simulink model "Chevrolet_PHEVmodel"  (R2024b)
settings: Solver=VariableStepAuto  StartTime=0.0  StopTime=10.0  RelTol=1e-3
undefined symbols (not defined in the file): automatic_gearbox, DiscIntNeverNeededParam, eta_EG_map, eta_EM_map, g, h, H_u, k_cs, P_aux, P_CE_cutoff, P_CE_idle, r, rho, rho_f, T_CE_cutoff, T_CE_max, T_EG_max, T_EM_max, theta_CE, theta_EM, V_CE_map, w_CE_idle, w_CE_max, w_CE_upper, w_EG_row, w_EG_upper, w_EM_row, w_EM_upper
(part 1 of 2)
settings Model: Creator=Imane  LastModifiedBy=Imane

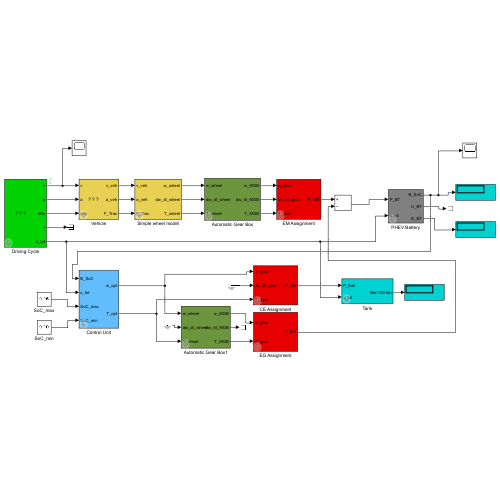
[thumbnail: Simulink's stored preview of the top-level diagram]
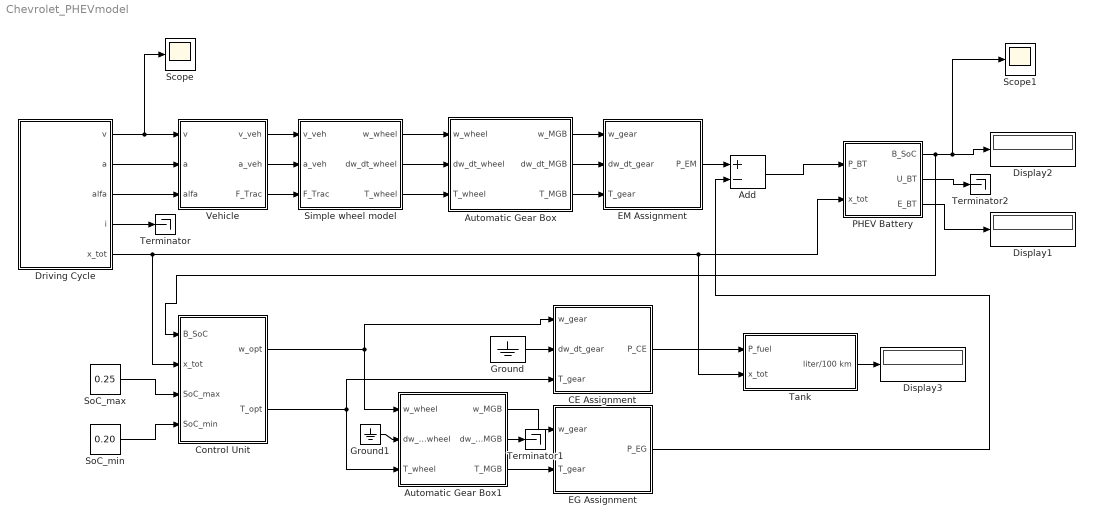
== system Chevrolet_PHEVmodel ==
  Add : Sum  Inputs=+-
  Automatic Gear Box : Subsystem  Tag=transmission  mask(Automatic Gear Box){nog=1, i=[1], i_diff=5, gearon=[], gearoff=[], d=0.62, e_GT=0.98, P_GT0=300, w_wheel_min=1}
      mask prompts: nog "Number of gears"; i "Gear ratio vector"; i_diff "Differential gear [-]"; gearon "Switching points for upshift [km/h]"; gearoff "Switching points for downshift [km/h]"; d "Wheel diameter"; e_GT "Efficiency [-]"; P_GT0 "Idling losses (friction) [W]"; w_wheel_min "Minimum wheel speed beyond which losses are generated [rad/s]"
      mask help:
      | This block simulates a automatic gear box, can handle up to 16 gears.
      |
      | Input:
      | =====
      | 	w_wheel	Speed of the wheel [rad/s]
      | 	dw_dt_wheel	Acceleration of the wheel [rad/s^2],
      | 	T_wheel	Torque on the wheel [Nm]
      | 	i	Gear number [-]
      |
      | Output:
      | ======
      | 	w_MGB	Speed of the fly wheel [rad/s]
      | 	dw_dt_MGB	Acceleration of the fly wheel [rad/s^2]
      | 	T_MGB	Torque on the fly wheel [Nm]
      |
      | Number of gears:
      | ======
      | Specify the number of forward gears
      |
      | Shifting points for upshift:
      | ======
      | Vector specifying the velocity for shifting
      | [first_to_second_gear    second_to_third_gear    ....]
      | The number of elements in the vector should be Number of gears - 1.
      |
      | Shifting points for udownshift:
      | ======
      | Simular to upshift
      | [second_to_first_gear    third_to_second_gear    ....]
      mask init:
      | init_AGB;
  Automatic Gear Box1 : Subsystem  Tag=transmission  mask(Automatic Gear Box){nog=1, i=[1], i_diff=1, gearon=[], gearoff=[], d=0.62, e_GT=0.98, P_GT0=0, w_wheel_min=1}
      mask prompts: nog "Number of gears"; i "Gear ratio vector"; i_diff "Differential gear [-]"; gearon "Switching points for upshift [km/h]"; gearoff "Switching points for downshift [km/h]"; d "Wheel diameter"; e_GT "Efficiency [-]"; P_GT0 "Idling losses (friction) [W]"; w_wheel_min "Minimum wheel speed beyond which losses are generated [rad/s]"
      mask help:
      | This block simulates a automatic gear box, can handle up to 16 gears.
      |
      | Input:
      | =====
      | 	w_wheel	Speed of the wheel [rad/s]
      | 	dw_dt_wheel	Acceleration of the wheel [rad/s^2],
      | 	T_wheel	Torque on the wheel [Nm]
      | 	i	Gear number [-]
      |
      | Output:
      | ======
      | 	w_MGB	Speed of the fly wheel [rad/s]
      | 	dw_dt_MGB	Acceleration of the fly wheel [rad/s^2]
      | 	T_MGB	Torque on the fly wheel [Nm]
      |
      | Number of gears:
      | ======
      | Specify the number of forward gears
      |
      | Shifting points for upshift:
      | ======
      | Vector specifying the velocity for shifting
      | [first_to_second_gear    second_to_third_gear    ....]
      | The number of elements in the vector should be Number of gears - 1.
      |
      | Shifting points for udownshift:
      | ======
      | Simular to upshift
      | [second_to_first_gear    third_to_second_gear    ....]
      mask init:
      | init_AGB;
  CE Assignment : Subsystem  Tag=combustion engine  mask(Combustion Engine (based on consumption map)){engine_type=Gasoline, P_ice=25, ENABLE_FUEL_CUTOFF=on}
      mask prompts: engine_type "Engine type"; P_ice "Power [kW]"; ENABLE_FUEL_CUTOFF "Enable fuel cutoff"
      mask help:
      | This block simulates the behaviour of a combustion engine. The block is based on consumption maps for medium sized passenger cars.
      |
      | NA Gasoline:
      | max power @ 5000 rpm
      | max torque @ 3000 rpm
      |
      | Small Diesel:
      | max power @ 4500 rpm
      | max torque @ 2000 rpm
      |
      | Large Diesel:
      | max power @ 1500 rpm
      | max torque @ 1500 rpm
      |
      |
      | Input:
      | =====
      | 	w_gear	Speed of the fly wheel [rad/s]
      | 	dw_dt_gear	Acceleration of the fly wheel [rad/s^2]
      | 	T_gear	Torque on the fly wheel [Nm]
      |
      | Output:
      | ======
      | 	P_CE	Fuel power consumed by the combustion engine [W]
      mask init:
      | init_AssCE_map;
      mask TypeOptions engine_type: Gasoline | Small Diesel | Large Diesel
  "Control Unit " : Subsystem  Tag=control unit  mask(Control Unit){}
      mask help:
      | This block gives the user the opportunity to design his/her own control unit.
      |
      | The user can define the inputs and outputs  by himself/herself.
  Display1 : Display
  Display2 : Display
  Display3 : Display
  Driving Cycle : Subsystem  Tag=cycle  mask(Driving Cycle){cyclename1=NEDC, stepsize=1, autostop=on}
      mask prompts: cyclename1 "Choose a cycle"; stepsize "Step size [s]"; autostop "Enable automatic simulation stop"
      mask help:
      | This block loads the cycle data such as time, speed, acceleration and gear number,  from the specified data file and makes it available on the output of the cycle block.
      |
      | Output:
      | ======
      | 	v	Speed [m/s]
      | 	a	Acceleration [m/s^2]
      | 	i	Gear number [-]
      | 	x_tot	Total distance [m]
      |
      | Tip:
      | ===
      | Probably you don't need the gear number "i". If so you can terminate
      | it with a "Terminator" out of the "Simulink Library/Connections."
      |
      | Driving cycle:
      | ===
      | Select a driving cycle from the list below or specify your own (place your .mat file in the
      | directory Data/DrivingCycles/UserDefined)
      |
      | ECE_MAN
      | ECE_R15s
      | EUDC
      | EUDC_MAN
      | City
      | City_MAN
      | NEDC
      | NEDC_MANl
      | GOT1
      | GOT2
      | GOT3
      | 10_15_MODE
      | 10_MODE
      | 10_MODE_3
      | 11_MODE
      | 11_MODE_4
      | 15_MODE
      | City_I
      | City_II
      | FTP_75
      | FTP_Highway
      |
      | WLTC
      | RTS95
      |
      |
      | Step size:
      | ========
      | Default value is 1. Don't change it, unless you are familiar with the programs of the QSS TB.
      |
      | Enable automatic simulation stop:
      | ===========================
      | Stops the simulation automatically at the end of the cycle.
      | Be careful: If you have a component in your model that has to run after the cycle has finished, e.g. a battery to charge, remove the mark!
      mask init:
      | init_driving_cycle1;
      mask Display: plot(T_zplot, V_zplot);
  EG Assignment : Subsystem  mask(Electric Generator){P_eg=15}
      mask prompts: P_eg "Maximum mechanical power [kW]"
      mask help:
      | This block simulates the behaviour of an electric generator. The block is based on an efficiency map.
      |
      | Input:
      | =====
      | 	w_gear	Speed of the generator [rad/s]
      | 	T_gear	Torque of the generator [Nm]
      |
      | Output:
      | ======
      | 	P_EG	Electric power of the generator [W]
      |
      | Generator map:
      | ======
      | The generator map file must contain the following variables:
      | eta_EG_map		% Efficiency map                    [-]
      | w_EG_row                        % Generator speed range             [rad/s]
      | T_EG_col		% Generator torque range            [Nm]
      | w_EG_max		% Maximum generator speed           [rad/s]
      | T_EG_max		% Maximum generator torque          [Nm]
      |
      | ======
      mask init:
      | init_EG_ass;
  EM Assignment : Subsystem  mask(Electric Motor){P_em=90}
      mask prompts: P_em "Power [kW]"
      mask help:
      | This block simulates the behaviour of an electric motor. The block is based on an efficiency map. The map is located in the Data/EnergyConvertter/ElectricMotor directory.
      |
      | Maximum speed och the electric motor is 6000 rpm
      | Field weakening region starts at 1500 rpm
      | Maximum mechanical power is at 2150 rpm
      | The maximum torque is 5.98 Nm/kW multiplied with the power you select.
      |
      | Input:
      | =====
      | 	w_gear	Speed of the motor [rad/s]
      | 	dw_dt_gear	Acceleration of the motor [rad/s^2]
      | 	T_gear	Torque of the motor [Nm]
      |
      | Output:
      | ======
      | 	P_EM	Electric Power consumed by the  motor [W]
      mask init:
      | init_EM_ass;
  Ground : Ground
  Ground1 : Ground
  PHEV Battery : Subsystem  Tag=battery  mask(Battery){cell_series=100, cell_parallel=1, Q_BT_IC_rel=25}
      mask prompts: cell_series "Number of series cells"; cell_parallel "Number  of parallel cells"; Q_BT_IC_rel "Initial charge of battery [%]"
      mask help:
      | This block simulates a PHEV battery.
      | The open circuit voltage and resistance depend on the battery state of charge.
      | Open circuit voltage is dependent on how many batteries that are connected in series
      | Each cell has a capacity of 35 Ah and the cell open-circuit voltage is 3.8 V at 50% SoC.
      | Max peak current per cell is +/- 200 A
      |
      | Input:
      | =====
      | 	P_BT	Power from/to the battery [W]
      | 		P_BT < 0: battery charging
      | 		P_BT > 0: battery discharging
      | 	x_tot	Total distance [m]
      |
      | Output:
      | ======
      | 	B_SoC	State of charge ratio [-]
      | 	U_BT	Voltage of the battery [V]
      | 	E_BT	Energy consumption [kWh/100 km]
      mask init:
      | init_BT_Assign;
  Scope : Scope
  Scope1 : Scope
  Simple wheel model : Subsystem  Tag=simple transmission  mask(Simple wheel model){d_wheel=0.62}
      mask prompts: d_wheel "Wheel diameter [m]"
      mask help:
      | This block simulates a simple wheel model without tire slip and no losses.
      |
      | Input:
      | =====
      | 	v_veh	Speed of the vehicle [m/s]
      | 	a_veh	Acceleration of the vehicle [m/s^2]
      | 	F_Trac	Traction force [N]
      |
      | Output:
      | ======
      | 	w_wheel		Speed of the wheel shaft [rad/s]
      | 	dw_dt_wheel		Acceleration of the wheel shaft [rad/s^2]
      | 	T_wheel		Torque on the wheel shaft [Nm]
  SoC_max : Constant  Value=0.25
  SoC_min : Constant  Value=0.20
  Tank : Subsystem  Tag=tank  mask(Tank){fuel=Diesel, flag_cold_start=on}
      mask prompts: flag_cold_start "Include cold start losses"
      mask help:
      | This block integrates the power (the fuel mass flow) required by the combustion engine or the fuel cell and calculates the energy consumption in liter/100 km.
      |
      | Input:
      | =====
      | 	P_fuel	Power (fuel mass flow) required [W]
      | 	x_tot	Total distance [m]
      |
      | Output:
      | ======
      | 	V	Fuel consumption [liter/100 km]
      mask init:
      | init_tank;
      mask TypeOptions fuel: Gasoline | Diesel | Hydrogen
  Terminator : Terminator
  Terminator1 : Terminator
  Terminator2 : Terminator
  Vehicle : Subsystem  Tag=vehicle  mask(Vehicle){m_f=1250+80+100+200, A_f=2.1, cw=0.27, mu=0.009, k_inertia=4}
      mask prompts: m_f "Total mass of the vehicle [kg]"; A_f "Vehicle cross section [m^2]"; cw "Drag coefficient [-]"; mu "Rolling resistance coefficient [-]"; k_inertia "Mass increase due to Rotating inertia [%]"
      mask help:
      | This block computes the force required by the vehicle.
      |
      | Input:
      | =====
      | 	v	Speed [m/s]
      | 	a	Acceleration [m/s^2]
      |    	alfa    	Road inclination angle [rad]
      |
      | Output:
      | ======
      | 	v_veh	Speed of the vehicle [m/s]
      | 	a_veh	Acceleration of the vehicle [m/s^2]
      | 	F_Trac	Traction Force required from the powertrain [N]
      mask init:
      | init_vehicle;
      mask Display: image('batteri_icon2.jpeg');
  wires:
  Automatic Gear Box/1(w_MGB) -> EM Assignment/1(w_gear)
  CE Assignment/1(P_CE) -> Tank/1(P_fuel)
  Tank/1(liter/100 km) -> Display3/1
  Automatic Gear Box1/1(w_MGB) -> EG Assignment/1(w_gear)
  "Control Unit "/2(T_opt) -> CE Assignment/3(T_gear), Automatic Gear Box1/3(T_wheel)
  Vehicle/1(v_veh) -> Simple wheel model/1(v_veh)
  SoC_min/1 -> "Control Unit "/4(SoC_min)
  "Control Unit "/1(w_opt) -> CE Assignment/1(w_gear), Automatic Gear Box1/1(w_wheel)
  Automatic Gear Box/3(T_MGB) -> EM Assignment/3(T_gear)
  PHEV Battery/3(E_BT) -> Display1/1
  Simple wheel model/2(dw_dt_wheel) -> Automatic Gear Box/2(dw_dt_wheel)
  Ground/1 -> CE Assignment/2(dw_dt_gear)
  EM Assignment/1(P_EM) -> Add/1
  Simple wheel model/3(T_wheel) -> Automatic Gear Box/3(T_wheel)
  EG Assignment/1(P_EG) -> Add/2
  Driving Cycle/4(i) -> Terminator/1
  PHEV Battery/2(U_BT) -> Terminator2/1
  Driving Cycle/2(a) -> Vehicle/2(a)
  Driving Cycle/1(v) -> Scope/1, Vehicle/1(v)
  SoC_max/1 -> "Control Unit "/3(SoC_max)
  Automatic Gear Box1/3(T_MGB) -> EG Assignment/2(T_gear)
  Ground1/1 -> Automatic Gear Box1/2(dw_dt_wheel)
  Vehicle/2(a_veh) -> Simple wheel model/2(a_veh)
  PHEV Battery/1(B_SoC) -> "Control Unit "/1(B_SoC), Display2/1, Scope1/1
  Vehicle/3(F_Trac) -> Simple wheel model/3(F_Trac)
  Driving Cycle/5(x_tot) -> "Control Unit "/2(x_tot), Tank/2(x_tot), PHEV Battery/2(x_tot)
  Automatic Gear Box/2(dw_dt_MGB) -> EM Assignment/2(dw_dt_gear)
  Driving Cycle/3(alfa) -> Vehicle/3(alfa)
  Automatic Gear Box1/2(dw_dt_MGB) -> Terminator1/1
  Simple wheel model/1(w_wheel) -> Automatic Gear Box/1(w_wheel)
  Add/1 -> PHEV Battery/1(P_BT)

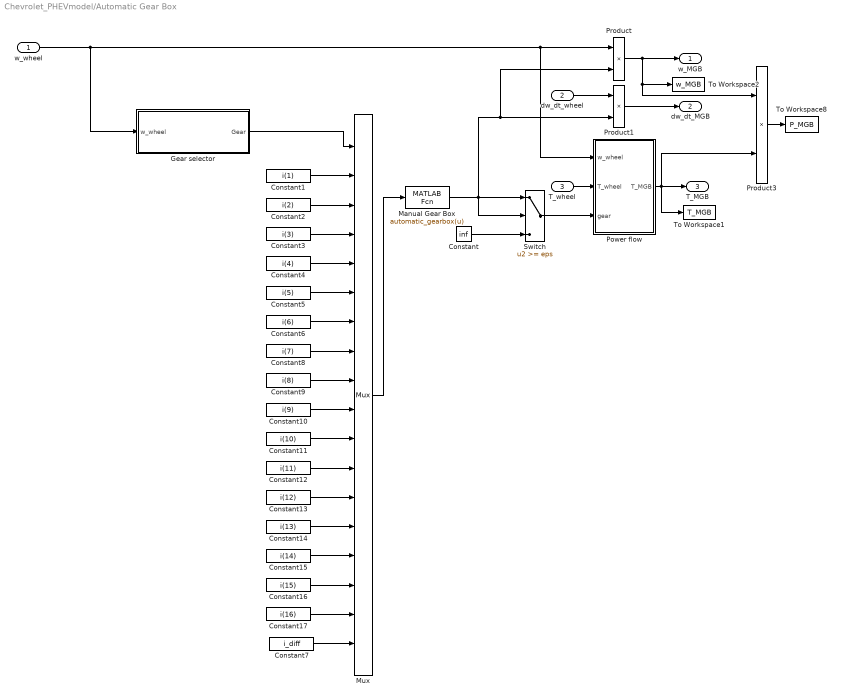
== system Chevrolet_PHEVmodel/Automatic Gear Box ==
  w_wheel : Inport
  dw_dt_wheel : Inport  Port=2
  T_wheel : Inport  Port=3
  Constant : Constant  Value=inf
  Constant1 : Constant  Value=i(1)
  Constant10 : Constant  Value=i(9)
  Constant11 : Constant  Value=i(10)
  Constant12 : Constant  Value=i(11)
  Constant13 : Constant  Value=i(12)
  Constant14 : Constant  Value=i(13)
  Constant15 : Constant  Value=i(14)
  Constant16 : Constant  Value=i(15)
  Constant17 : Constant  Value=i(16)
  Constant2 : Constant  Value=i(2)
  Constant3 : Constant  Value=i(3)
  Constant4 : Constant  Value=i(4)
  Constant5 : Constant  Value=i(5)
  Constant6 : Constant  Value=i(6)
  Constant7 : Constant  Value=i_diff
  Constant8 : Constant  Value=i(7)
  Constant9 : Constant  Value=i(8)
  Gear selector : Subsystem
  Manual Gear Box : MATLABFcn  MATLABFcn=automatic_gearbox(u)  OutputDimensions=1
  Mux : Mux  Inputs=18
  Power flow : Subsystem
  Product : Product  InputSameDT=on  RndMeth=Zero  SaturateOnIntegerOverflow=on  OutDataTypeStr=Inherit: Same as first input
  Product1 : Product  InputSameDT=on  RndMeth=Zero  SaturateOnIntegerOverflow=on  OutDataTypeStr=Inherit: Same as first input
  Product3 : Product  InputSameDT=on  RndMeth=Zero  SaturateOnIntegerOverflow=on  OutDataTypeStr=Inherit: Same as first input
  Switch : Switch  Threshold=eps
  To Workspace1 : ToWorkspace  VariableName=T_MGB  SampleTime=-1
  To Workspace2 : ToWorkspace  VariableName=w_MGB  SampleTime=-1
  To Workspace8 : ToWorkspace  VariableName=P_MGB  SampleTime=-1
  w_MGB : Outport  InitialOutput=0
  dw_dt_MGB : Outport  Port=2  InitialOutput=0
  T_MGB : Outport  Port=3  InitialOutput=0
  wires:
  Constant17/1 -> Mux/17
  Constant16/1 -> Mux/16
  Constant15/1 -> Mux/15
  Constant14/1 -> Mux/14
  Constant13/1 -> Mux/13
  Constant12/1 -> Mux/12
  Constant11/1 -> Mux/11
  Constant10/1 -> Mux/10
  Constant9/1 -> Mux/9
  Constant8/1 -> Mux/8
  Constant7/1 -> Mux/18
  Power flow/1(T_MGB) -> T_MGB/1, Product3/2, To Workspace1/1
  Product/1 -> w_MGB/1, Product3/1, To Workspace2/1
  Constant/1 -> Switch/3
  w_wheel/1 -> Gear selector/1(w_wheel), Product/1, Power flow/1(w_wheel)
  Product1/1 -> dw_dt_MGB/1
  dw_dt_wheel/1 -> Product1/1
  Manual Gear Box/1 -> Product/2, Product1/2, Switch/2, Switch/1
  Product3/1 -> To Workspace8/1
  Switch/1 -> Power flow/3(gear)
  T_wheel/1 -> Power flow/2(T_wheel)
  Constant1/1 -> Mux/2
  Constant2/1 -> Mux/3
  Constant3/1 -> Mux/4
  Constant4/1 -> Mux/5
  Constant5/1 -> Mux/6
  Constant6/1 -> Mux/7
  Gear selector/1(Gear) -> Mux/1
  Mux/1 -> Manual Gear Box/1

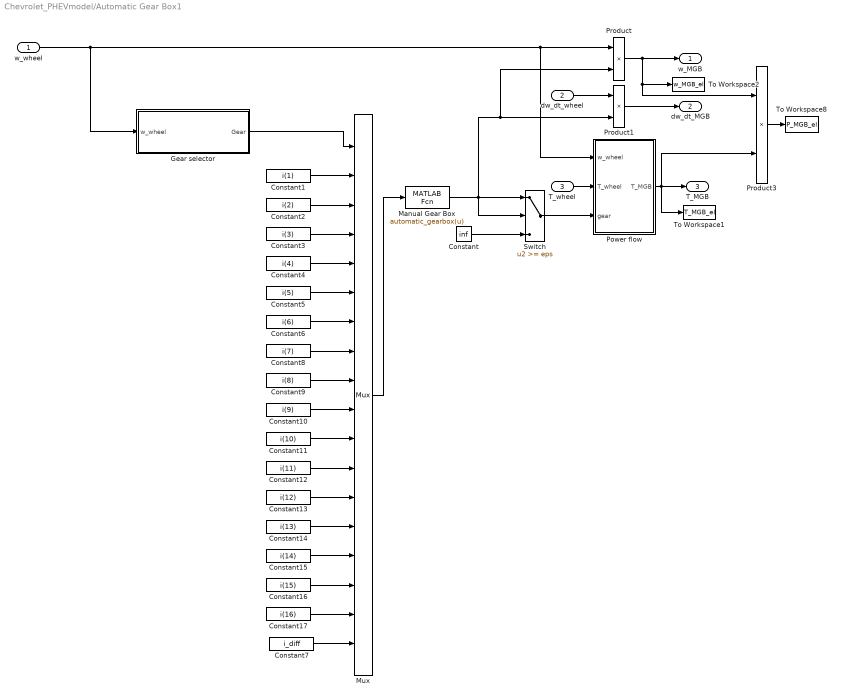
== system Chevrolet_PHEVmodel/Automatic Gear Box1 ==
  w_wheel : Inport
  dw_dt_wheel : Inport  Port=2
  T_wheel : Inport  Port=3
  Constant : Constant  Value=inf
  Constant1 : Constant  Value=i(1)
  Constant10 : Constant  Value=i(9)
  Constant11 : Constant  Value=i(10)
  Constant12 : Constant  Value=i(11)
  Constant13 : Constant  Value=i(12)
  Constant14 : Constant  Value=i(13)
  Constant15 : Constant  Value=i(14)
  Constant16 : Constant  Value=i(15)
  Constant17 : Constant  Value=i(16)
  Constant2 : Constant  Value=i(2)
  Constant3 : Constant  Value=i(3)
  Constant4 : Constant  Value=i(4)
  Constant5 : Constant  Value=i(5)
  Constant6 : Constant  Value=i(6)
  Constant7 : Constant  Value=i_diff
  Constant8 : Constant  Value=i(7)
  Constant9 : Constant  Value=i(8)
  Gear selector : Subsystem
  Manual Gear Box : MATLABFcn  MATLABFcn=automatic_gearbox(u)  OutputDimensions=1
  Mux : Mux  Inputs=18
  Power flow : Subsystem
  Product : Product  InputSameDT=on  RndMeth=Zero  SaturateOnIntegerOverflow=on  OutDataTypeStr=Inherit: Same as first input
  Product1 : Product  InputSameDT=on  RndMeth=Zero  SaturateOnIntegerOverflow=on  OutDataTypeStr=Inherit: Same as first input
  Product3 : Product  InputSameDT=on  RndMeth=Zero  SaturateOnIntegerOverflow=on  OutDataTypeStr=Inherit: Same as first input
  Switch : Switch  Threshold=eps
  To Workspace1 : ToWorkspace  VariableName=T_MGB_el  SampleTime=-1
  To Workspace2 : ToWorkspace  VariableName=w_MGB_el  SampleTime=-1
  To Workspace8 : ToWorkspace  VariableName=P_MGB_el  SampleTime=-1
  w_MGB : Outport  InitialOutput=0
  dw_dt_MGB : Outport  Port=2  InitialOutput=0
  T_MGB : Outport  Port=3  InitialOutput=0
  wires:
  Constant17/1 -> Mux/17
  Constant16/1 -> Mux/16
  Constant15/1 -> Mux/15
  Constant14/1 -> Mux/14
  Constant13/1 -> Mux/13
  Constant12/1 -> Mux/12
  Constant11/1 -> Mux/11
  Constant10/1 -> Mux/10
  Constant9/1 -> Mux/9
  Constant8/1 -> Mux/8
  Constant7/1 -> Mux/18
  Power flow/1(T_MGB) -> T_MGB/1, Product3/2, To Workspace1/1
  Product/1 -> w_MGB/1, Product3/1, To Workspace2/1
  Constant/1 -> Switch/3
  w_wheel/1 -> Gear selector/1(w_wheel), Product/1, Power flow/1(w_wheel)
  Product1/1 -> dw_dt_MGB/1
  dw_dt_wheel/1 -> Product1/1
  Manual Gear Box/1 -> Product/2, Product1/2, Switch/2, Switch/1
  Product3/1 -> To Workspace8/1
  Switch/1 -> Power flow/3(gear)
  T_wheel/1 -> Power flow/2(T_wheel)
  Constant1/1 -> Mux/2
  Constant2/1 -> Mux/3
  Constant3/1 -> Mux/4
  Constant4/1 -> Mux/5
  Constant5/1 -> Mux/6
  Constant6/1 -> Mux/7
  Gear selector/1(Gear) -> Mux/1
  Mux/1 -> Manual Gear Box/1

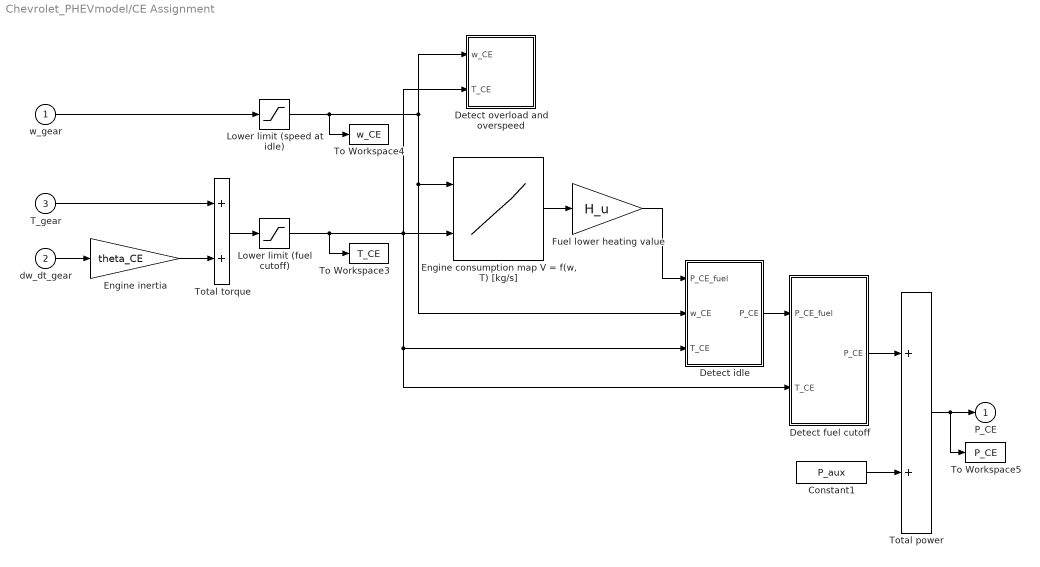
== system Chevrolet_PHEVmodel/CE Assignment ==
  w_gear : Inport
  dw_dt_gear : Inport  Port=2
  T_gear : Inport  Port=3
  Constant1 : Constant  Value=P_aux
  Detect fuel cutoff : Subsystem
  Detect idle : Subsystem
  Detect overload and overspeed : Subsystem
  "Engine consumption map V = f(w, T) [kg/s]" : Lookup2D  RowIndex=w_CE_row  ColumnIndex=T_CE_col  Table=V_CE_map  SaturateOnIntegerOverflow=off  InputSameDT=off
  Engine inertia : Gain  Gain=theta_CE  SaturateOnIntegerOverflow=on  OutDataTypeStr=Inherit: Same as input  ParamDataTypeStr=Inherit: Same as input
  Fuel lower heating value : Gain  Gain=H_u  SaturateOnIntegerOverflow=on  OutDataTypeStr=Inherit: Same as input  ParamDataTypeStr=Inherit: Same as input
  Lower limit (fuel cutoff) : Saturate  UpperLimit=inf  LowerLimit=T_CE_cutoff
  Lower limit (speed at idle) : Saturate  UpperLimit=inf  LowerLimit=w_CE_idle
  To Workspace3 : ToWorkspace  VariableName=T_CE  SampleTime=-1
  To Workspace4 : ToWorkspace  VariableName=w_CE  SampleTime=-1
  To Workspace5 : ToWorkspace  VariableName=P_CE  SampleTime=-1
  Total power : Sum  InputSameDT=on  SaturateOnIntegerOverflow=on  OutDataTypeStr=Inherit: Same as first input
  Total torque : Sum  InputSameDT=on  SaturateOnIntegerOverflow=on  OutDataTypeStr=Inherit: Same as first input
  P_CE : Outport  InitialOutput=0
  wires:
  T_gear/1 -> Total torque/1
  dw_dt_gear/1 -> Engine inertia/1
  Total torque/1 -> Lower limit (fuel cutoff)/1
  Engine inertia/1 -> Total torque/2
  Lower limit (speed at idle)/1 -> Detect overload and overspeed/1(w_CE), Detect idle/2(w_CE), "Engine consumption map V = f(w, T) [kg/s]"/1, To Workspace4/1
  w_gear/1 -> Lower limit (speed at idle)/1
  Fuel lower heating value/1 -> Detect idle/1(P_CE_fuel)
  Detect idle/1(P_CE) -> Detect fuel cutoff/1(P_CE_fuel)
  "Engine consumption map V = f(w, T) [kg/s]"/1 -> Fuel lower heating value/1
  Detect fuel cutoff/1(P_CE) -> Total power/1
  Total power/1 -> P_CE/1, To Workspace5/1
  Constant1/1 -> Total power/2
  Lower limit (fuel cutoff)/1 -> Detect overload and overspeed/2(T_CE), "Engine consumption map V = f(w, T) [kg/s]"/2, Detect idle/3(T_CE), Detect fuel cutoff/2(T_CE), To Workspace3/1

== system Chevrolet_PHEVmodel/Control Unit  ==
  B_SoC : Inport
  x_tot : Inport  Port=2
  SoC_max : Inport  Port=3
  SoC_min : Inport  Port=4
  Gain : Gain  Gain=2500/60*2*pi
  Gain1 : Gain  Gain=40
  MATLAB Function : MATLAB Function  TreatAsAtomicUnit=on
  Memory : Memory
  w_opt : Outport  InitialOutput=0
  T_opt : Outport  Port=2  InitialOutput=0
  wires:
  x_tot/1 -> MATLAB Function/2(x_tot)
  B_SoC/1 -> MATLAB Function/1(B_SoC)
  Gain1/1 -> T_opt/1
  Gain/1 -> w_opt/1
  SoC_max/1 -> MATLAB Function/3(SoC_max)
  SoC_min/1 -> MATLAB Function/4(SoC_min)
  Memory/1 -> MATLAB Function/5(u_previous)
  MATLAB Function/1(y) -> Gain1/1, Gain/1, Memory/1

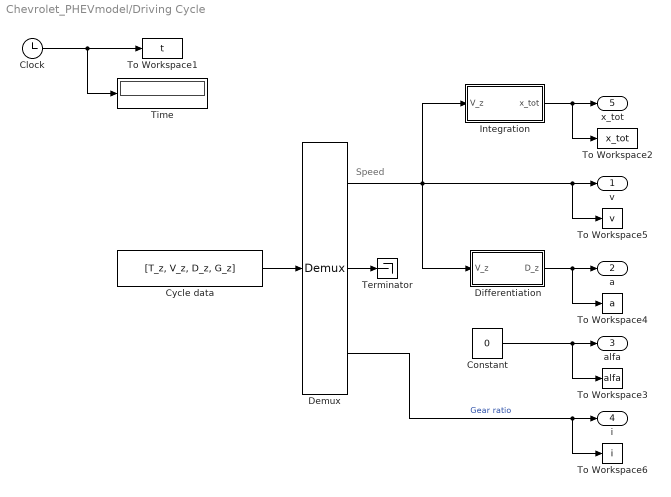
== system Chevrolet_PHEVmodel/Driving Cycle ==
  note: Speed
  Clock : Clock
  Constant : Constant  Value=0
  Cycle data : FromWorkspace  VariableName=[T_z, V_z, D_z, G_z]  SampleTime=h  ZeroCross=off
  Demux : Demux  Outputs=3
      settings: DisplayOption=none
  Differentiation : Subsystem
  Integration : Subsystem
  Terminator : Terminator
  Time : Display
  To Workspace1 : ToWorkspace  VariableName=t  SampleTime=-1
  To Workspace2 : ToWorkspace  VariableName=x_tot  SampleTime=-1
  To Workspace3 : ToWorkspace  VariableName=alfa  SampleTime=-1
  To Workspace4 : ToWorkspace  VariableName=a  SampleTime=-1
  To Workspace5 : ToWorkspace  VariableName=v  SampleTime=-1
  To Workspace6 : ToWorkspace  VariableName=i  SampleTime=-1
  v : Outport  InitialOutput=0
  a : Outport  Port=2  InitialOutput=0
  alfa : Outport  Port=3  InitialOutput=0
  i : Outport  Port=4  InitialOutput=0
  x_tot : Outport  Port=5  InitialOutput=0
  wires:
  Demux/1 -> Integration/1(V_z), Differentiation/1(V_z), v/1, To Workspace5/1
  Cycle data/1 -> Demux/1
  Differentiation/1(D_z) -> To Workspace4/1, a/1
  Demux/2 -> Terminator/1
  Integration/1(x_tot) -> x_tot/1, To Workspace2/1
  Demux/3 -> i/1, To Workspace6/1  "Gear ratio"
  Clock/1 -> Time/1, To Workspace1/1
  Constant/1 -> To Workspace3/1, alfa/1

== system Chevrolet_PHEVmodel/EG Assignment ==
  w_gear : Inport
  T_gear : Inport  Port=2
  Detect overload and overspeed : Subsystem
  "Efficiency eta = f(w, T)" : Lookup2D  RowIndex=w_EG_row  ColumnIndex=T_EG_col  Table=eta_EG_map  SaturateOnIntegerOverflow=off  InputSameDT=off
  Product : Product  Inputs=3  InputSameDT=on  RndMeth=Zero  SaturateOnIntegerOverflow=on  OutDataTypeStr=Inherit: Same as first input
  To Workspace1 : ToWorkspace  VariableName=w_EG  SampleTime=-1
  To Workspace2 : ToWorkspace  VariableName=T_EG  SampleTime=-1
  To Workspace5 : ToWorkspace  VariableName=P_EG  SampleTime=-1
  P_EG : Outport  InitialOutput=0
  wires:
  w_gear/1 -> To Workspace1/1, Detect overload and overspeed/1(w_EG), "Efficiency eta = f(w, T)"/1, Product/3
  Product/1 -> To Workspace5/1, P_EG/1
  "Efficiency eta = f(w, T)"/1 -> Product/1
  T_gear/1 -> To Workspace2/1, Detect overload and overspeed/2(T_EG), "Efficiency eta = f(w, T)"/2, Product/2

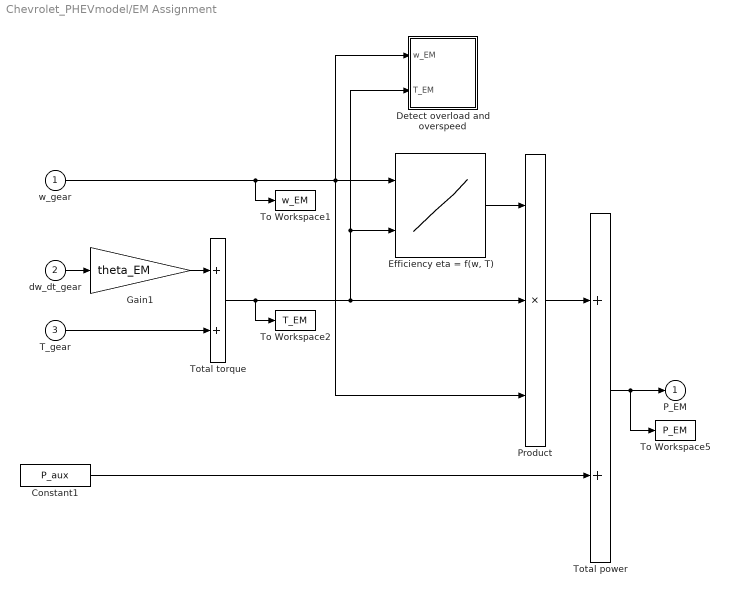
== system Chevrolet_PHEVmodel/EM Assignment ==
  w_gear : Inport
  dw_dt_gear : Inport  Port=2
  T_gear : Inport  Port=3
  Constant1 : Constant  Value=P_aux
  Detect overload and overspeed : Subsystem
  "Efficiency eta = f(w, T)" : Lookup2D  RowIndex=w_EM_row  ColumnIndex=T_EM_col  Table=eta_EM_map  SaturateOnIntegerOverflow=off  InputSameDT=off
  Gain1 : Gain  Gain=theta_EM  SaturateOnIntegerOverflow=on  OutDataTypeStr=Inherit: Same as input  ParamDataTypeStr=Inherit: Same as input
  Product : Product  Inputs=3  InputSameDT=on  RndMeth=Zero  SaturateOnIntegerOverflow=on  OutDataTypeStr=Inherit: Same as first input
  To Workspace1 : ToWorkspace  VariableName=w_EM  SampleTime=-1
  To Workspace2 : ToWorkspace  VariableName=T_EM  SampleTime=-1
  To Workspace5 : ToWorkspace  VariableName=P_EM  SampleTime=-1
  Total power : Sum  InputSameDT=on  SaturateOnIntegerOverflow=on  OutDataTypeStr=Inherit: Same as first input
  Total torque : Sum  InputSameDT=on  SaturateOnIntegerOverflow=on  OutDataTypeStr=Inherit: Same as first input
  P_EM : Outport  InitialOutput=0
  wires:
  Total power/1 -> To Workspace5/1, P_EM/1
  Product/1 -> Total power/1
  Constant1/1 -> Total power/2
  Total torque/1 -> To Workspace2/1, Product/2, "Efficiency eta = f(w, T)"/2, Detect overload and overspeed/2(T_EM)
  Gain1/1 -> Total torque/1
  T_gear/1 -> Total torque/2
  dw_dt_gear/1 -> Gain1/1
  "Efficiency eta = f(w, T)"/1 -> Product/1
  w_gear/1 -> To Workspace1/1, Product/3, "Efficiency eta = f(w, T)"/1, Detect overload and overspeed/1(w_EM)

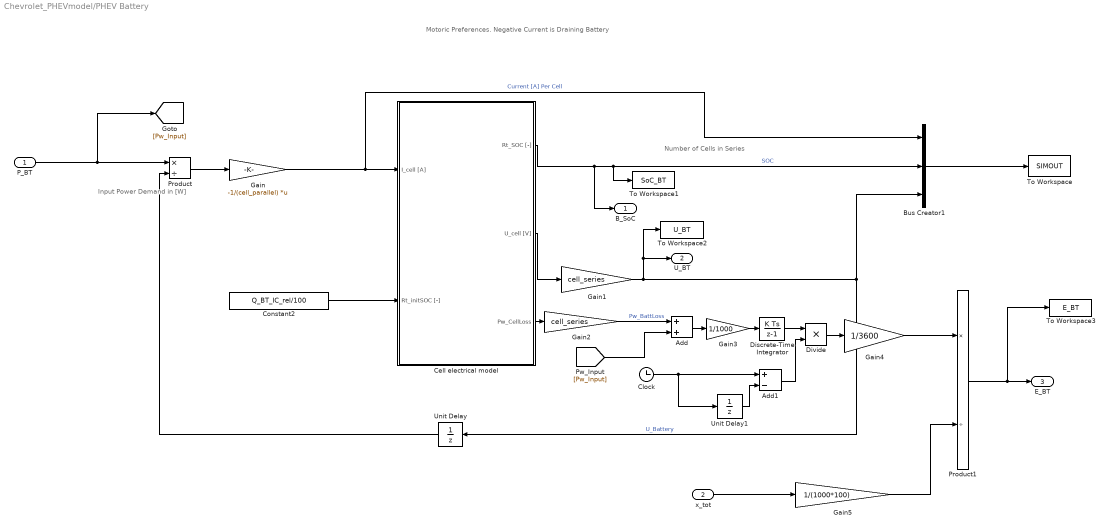
== system Chevrolet_PHEVmodel/PHEV Battery ==
  note: Input Power Demand in [W]
  note: Motoric Preferences. Negative Current is Draining Battery
  note: Number of Cells in Series
  P_BT : Inport
  x_tot : Inport  Port=2
  Add : Sum
  Add1 : Sum  Inputs=+-
  Bus Creator1 : BusCreator  Inputs=3
  Cell electrical model : Subsystem
  Clock : Clock
  Constant2 : Constant  Value=Q_BT_IC_rel/100
  Discrete-Time Integrator : DiscreteIntegrator  ICPrevOutput=DiscIntNeverNeededParam  ICPrevScaledInput=DiscIntNeverNeededParam
  Divide : Product  Inputs=**
  Gain : Gain  Gain=-1/(cell_parallel)  Multiplication=Matrix(K*u)
  Gain1 : Gain  Gain=cell_series
  Gain2 : Gain  Gain=cell_series
  Gain3 : Gain  Gain=1/1000
  Gain4 : Gain  Gain=1/3600
  Gain5 : Gain  Gain=1/(1000*100)
  Product : Product  Inputs=*/  RndMeth=Zero
  Product1 : Product  Inputs=*/  InputSameDT=on  RndMeth=Zero  SaturateOnIntegerOverflow=on  OutDataTypeStr=Inherit: Same as first input
  To Workspace : ToWorkspace  VariableName=SIMOUT  SaveFormat=Structure With Time  SampleTime=-1
  To Workspace1 : ToWorkspace  VariableName=SoC_BT  SampleTime=-1
      settings: RequirementInfo={} %GIDa_c6642060_f8db_4366_a618_aa68098668f7
  To Workspace2 : ToWorkspace  VariableName=U_BT  SampleTime=-1
      settings: RequirementInfo={} %GIDa_32590376_96d5_473d_a7bc_23059799ede8
  To Workspace3 : ToWorkspace  VariableName=E_BT  SampleTime=-1
  Unit Delay : UnitDelay  InitialCondition=4.07*cell_series  HasFrameUpgradeWarning=on
  Unit Delay1 : UnitDelay  HasFrameUpgradeWarning=on
  B_SoC : Outport  InitialOutput=0
  U_BT : Outport  Port=2  InitialOutput=0
  E_BT : Outport  Port=3  InitialOutput=0
  wires:
  Gain/1 -> Bus Creator1/1, Cell electrical model/1(I_cell [A])  "Current [A] Per Cell"
  Cell electrical model/2(U_cell [V]) -> Gain1/1
  Gain1/1 -> To Workspace2/1, U_BT/1, Bus Creator1/3, Unit Delay/1  "U_Battery"
  Constant2/1 -> Cell electrical model/2(Rt_initSOC [-])
  Product/1 -> Gain/1
  Unit Delay/1 -> Product/2
  Cell electrical model/1(Rt_SOC [-]) -> B_SoC/1, To Workspace1/1, Bus Creator1/2  "SOC"
  P_BT/1 -> [Pw_Input], Product/1
  Product1/1 -> To Workspace3/1, E_BT/1
  Cell electrical model/3(Pw_CellLoss) -> Gain2/1
  Gain2/1 -> Add/1  "Pw_BattLoss"
  [Pw_Input] -> Add/2
  Add/1 -> Gain3/1
  Gain3/1 -> Discrete-Time Integrator/1
  Divide/1 -> Gain4/1
  Gain4/1 -> Product1/1
  Gain5/1 -> Product1/2
  x_tot/1 -> Gain5/1
  Discrete-Time Integrator/1 -> Divide/1
  Bus Creator1/1 -> To Workspace/1
  Clock/1 -> Unit Delay1/1, Add1/1
  Unit Delay1/1 -> Add1/2
  Add1/1 -> Divide/2

== system Chevrolet_PHEVmodel/Simple wheel model ==
  v_veh : Inport
  a_veh : Inport  Port=2
  F_Trac : Inport  Port=3
  Gain1 : Gain  Gain=1/(0.5*d_wheel)  SaturateOnIntegerOverflow=on  OutDataTypeStr=Inherit: Same as input  ParamDataTypeStr=Inherit: Same as input
  Gain2 : Gain  Gain=1/(0.5*d_wheel)  SaturateOnIntegerOverflow=on  OutDataTypeStr=Inherit: Same as input  ParamDataTypeStr=Inherit: Same as input
  Gain3 : Gain  Gain=0.5*d_wheel  SaturateOnIntegerOverflow=on  OutDataTypeStr=Inherit: Same as input  ParamDataTypeStr=Inherit: Same as input
  To Workspace1 : ToWorkspace  VariableName=w_wheel  SampleTime=-1
  To Workspace2 : ToWorkspace  VariableName=T_wheel  SampleTime=-1
  To Workspace3 : ToWorkspace  VariableName=dw_dt_wheel  SampleTime=-1
  w_wheel : Outport  InitialOutput=0
  dw_dt_wheel : Outport  Port=2  InitialOutput=0
  T_wheel : Outport  Port=3  InitialOutput=0
  wires:
  v_veh/1 -> Gain1/1
  F_Trac/1 -> Gain3/1
  a_veh/1 -> Gain2/1
  Gain3/1 -> T_wheel/1, To Workspace2/1
  Gain1/1 -> To Workspace1/1, w_wheel/1
  Gain2/1 -> To Workspace3/1, dw_dt_wheel/1

== system Chevrolet_PHEVmodel/Tank ==
  P_fuel : Inport
  x_tot : Inport  Port=2
  Factor for cold start : Gain  Gain=k_cs  SaturateOnIntegerOverflow=on  OutDataTypeStr=Inherit: Same as input  ParamDataTypeStr=Inherit: Same as input
  Fu2131el density : Gain  Gain=1/rho_f  SaturateOnIntegerOverflow=on  OutDataTypeStr=Inherit: Same as input  ParamDataTypeStr=Inherit: Same as input
  Gain3 : Gain  Gain=1e5  SaturateOnIntegerOverflow=on  OutDataTypeStr=Inherit: Same as input  ParamDataTypeStr=Inherit: Same as input
  Integration : Subsystem
  Product : Product  Inputs=*/  InputSameDT=on  RndMeth=Zero  SaturateOnIntegerOverflow=on  OutDataTypeStr=Inherit: Same as first input
  To Workspace7 : ToWorkspace  VariableName=V_liter  SampleTime=-1
  liter/100 km : Outport  InitialOutput=0
  wires:
  Factor for cold start/1 -> Gain3/1
  Product/1 -> Factor for cold start/1
  Fu2131el density/1 -> Product/1
  Gain3/1 -> To Workspace7/1, liter/100 km/1
  Integration/1(m_fuel) -> Fu2131el density/1
  x_tot/1 -> Product/2
  P_fuel/1 -> Integration/1(P_fuel)

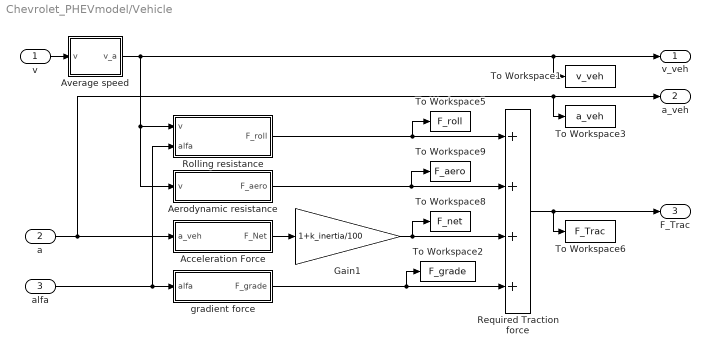
== system Chevrolet_PHEVmodel/Vehicle ==
  v : Inport
  a : Inport  Port=2
  alfa : Inport  Port=3
  Acceleration Force : Subsystem
  Aerodynamic resistance : Subsystem
  Average speed : Subsystem
  Gain1 : Gain  Gain=1+k_inertia/100  SaturateOnIntegerOverflow=on  OutDataTypeStr=Inherit: Same as input  ParamDataTypeStr=Inherit: Same as input
  Required Traction force : Sum  Inputs=++++  InputSameDT=on  SaturateOnIntegerOverflow=on  OutDataTypeStr=Inherit: Same as first input
  Rolling resistance : Subsystem
  To Workspace1 : ToWorkspace  VariableName=v_veh  SampleTime=-1
  To Workspace2 : ToWorkspace  VariableName=F_grade  SampleTime=-1
  To Workspace3 : ToWorkspace  VariableName=a_veh  SampleTime=-1
  To Workspace5 : ToWorkspace  VariableName=F_roll  SampleTime=-1
  To Workspace6 : ToWorkspace  VariableName=F_Trac  SampleTime=-1
  To Workspace8 : ToWorkspace  VariableName=F_net  SampleTime=-1
  To Workspace9 : ToWorkspace  VariableName=F_aero  SampleTime=-1
  gradient force : Subsystem
  v_veh : Outport  InitialOutput=0
  a_veh : Outport  Port=2  InitialOutput=0
  F_Trac : Outport  Port=3  InitialOutput=0
  wires:
  Average speed/1(v_a) -> To Workspace1/1, v_veh/1, Rolling resistance/1(v), Aerodynamic resistance/1(v)
  v/1 -> Average speed/1(v)
  a/1 -> a_veh/1, To Workspace3/1, Acceleration Force/1(a_veh)
  Rolling resistance/1(F_roll) -> Required Traction force/1, To Workspace5/1
  Aerodynamic resistance/1(F_aero) -> Required Traction force/2, To Workspace9/1
  Acceleration Force/1(F_Net) -> Gain1/1
  Required Traction force/1 -> To Workspace6/1, F_Trac/1
  alfa/1 -> Rolling resistance/2(alfa), gradient force/1(alfa)
  gradient force/1(F_grade) -> Required Traction force/4, To Workspace2/1
  Gain1/1 -> To Workspace8/1, Required Traction force/3

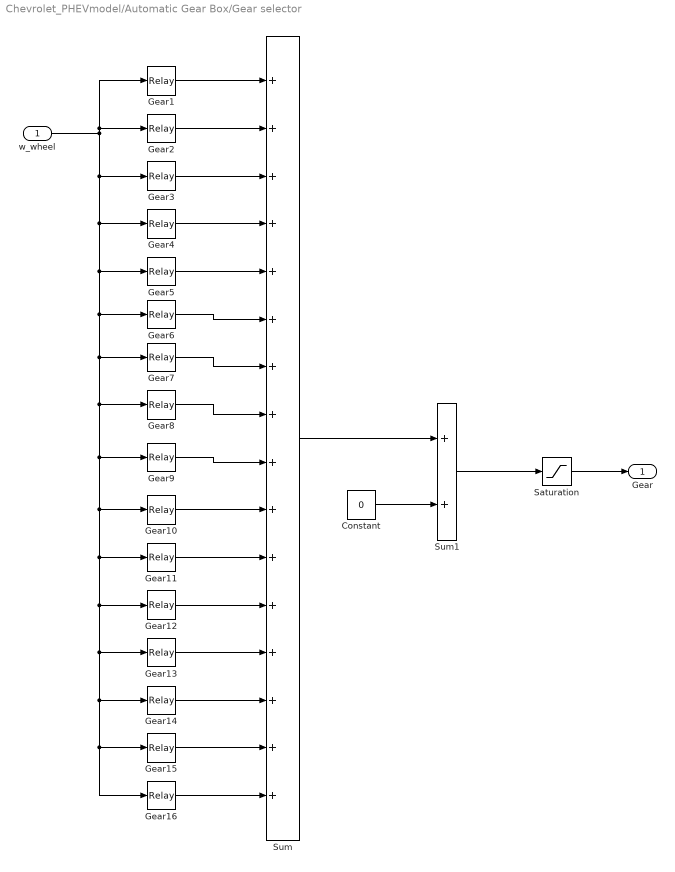
== system Chevrolet_PHEVmodel/Automatic Gear Box/Gear selector ==
  w_wheel : Inport
  Constant : Constant  Value=0
  Gear1 : Relay  OffSwitchValue=0
  Gear10 : Relay  OnSwitchValue=gearon(9)/3.6/r  OffSwitchValue=gearoff(9)/3.6/r
  Gear11 : Relay  OnSwitchValue=gearon(10)/3.6/r  OffSwitchValue=gearoff(10)/3.6/r
  Gear12 : Relay  OnSwitchValue=gearon(11)/3.6/r  OffSwitchValue=gearoff(11)/3.6/r
  Gear13 : Relay  OnSwitchValue=gearon(12)/3.6/r  OffSwitchValue=gearoff(12)/3.6/r
  Gear14 : Relay  OnSwitchValue=gearon(13)/3.6/r  OffSwitchValue=gearoff(13)/3.6/r
  Gear15 : Relay  OnSwitchValue=gearon(14)/3.6/r  OffSwitchValue=gearoff(14)/3.6/r
  Gear16 : Relay  OnSwitchValue=gearon(15)/3.6/r  OffSwitchValue=gearoff(15)/3.6/r
  Gear2 : Relay  OnSwitchValue=gearon(1)/3.6/r  OffSwitchValue=gearoff(1)/3.6/r
  Gear3 : Relay  OnSwitchValue=gearon(2)/3.6/r  OffSwitchValue=gearoff(2)/3.6/r
  Gear4 : Relay  OnSwitchValue=gearon(3)/3.6/r  OffSwitchValue=gearoff(3)/3.6/r
  Gear5 : Relay  OnSwitchValue=gearon(4)/3.6/r  OffSwitchValue=gearoff(4)/3.6/r
  Gear6 : Relay  OnSwitchValue=gearon(5)/3.6/r  OffSwitchValue=gearoff(5)/3.6/r
  Gear7 : Relay  OnSwitchValue=gearon(6)/3.6/r  OffSwitchValue=gearoff(6)/3.6/r
  Gear8 : Relay  OnSwitchValue=gearon(7)/3.6/r  OffSwitchValue=gearoff(7)/3.6/r
  Gear9 : Relay  OnSwitchValue=gearon(8)/3.6/r  OffSwitchValue=gearoff(8)/3.6/r
  Saturation : Saturate  UpperLimit=nog  LowerLimit=0
  Sum : Sum  Inputs=16  SaturateOnIntegerOverflow=on
  Sum1 : Sum  Inputs=2  SaturateOnIntegerOverflow=on
  Gear : Outport
  wires:
  Saturation/1 -> Gear/1
  Gear6/1 -> Sum/6
  Gear7/1 -> Sum/7
  Gear8/1 -> Sum/8
  Gear9/1 -> Sum/9
  Gear10/1 -> Sum/10
  Gear11/1 -> Sum/11
  Gear12/1 -> Sum/12
  Gear13/1 -> Sum/13
  Gear14/1 -> Sum/14
  Gear15/1 -> Sum/15
  Gear16/1 -> Sum/16
  Gear5/1 -> Sum/5
  w_wheel/1 -> Gear16/1, Gear15/1, Gear14/1, Gear13/1, Gear12/1, Gear11/1, Gear10/1, Gear9/1, Gear8/1, Gear7/1, Gear6/1, Gear5/1, Gear4/1, Gear3/1, Gear1/1, Gear2/1
  Gear1/1 -> Sum/1
  Gear2/1 -> Sum/2
  Gear3/1 -> Sum/3
  Gear4/1 -> Sum/4
  Sum/1 -> Sum1/1
  Sum1/1 -> Saturation/1
  Constant/1 -> Sum1/2

== system Chevrolet_PHEVmodel/Automatic Gear Box/Power flow ==
  w_wheel : Inport
  T_wheel : Inport  Port=2
  gear : Inport  Port=3
  "Engine -> Wheel" : Subsystem
  Switch1 : Switch
  "Wheel -> Engine" : Subsystem
  T_MGB : Outport  InitialOutput=0
  wires:
  w_wheel/1 -> "Wheel -> Engine"/1(w_wheel), "Engine -> Wheel"/1(w_wheel)
  gear/1 -> "Wheel -> Engine"/3(gear), "Engine -> Wheel"/3(gear)
  "Wheel -> Engine"/1(T_MGB-) -> Switch1/3
  T_wheel/1 -> "Wheel -> Engine"/2(T_wheel), "Engine -> Wheel"/2(T_wheel), Switch1/2
  "Engine -> Wheel"/1(T_MGB+) -> Switch1/1
  Switch1/1 -> T_MGB/1

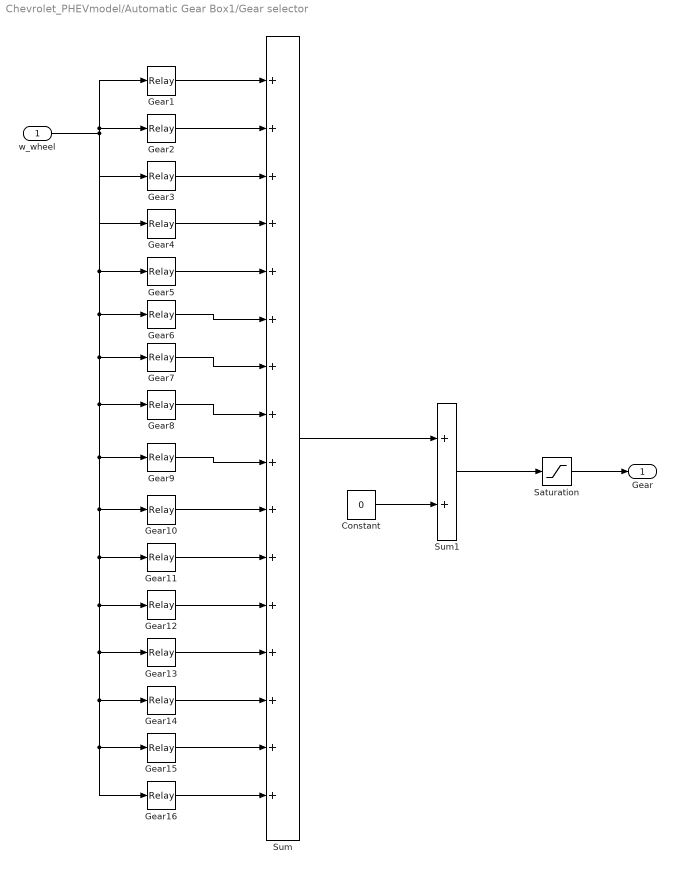
== system Chevrolet_PHEVmodel/Automatic Gear Box1/Gear selector ==
  w_wheel : Inport
  Constant : Constant  Value=0
  Gear1 : Relay  OffSwitchValue=0
  Gear10 : Relay  OnSwitchValue=gearon(9)/3.6/r  OffSwitchValue=gearoff(9)/3.6/r
  Gear11 : Relay  OnSwitchValue=gearon(10)/3.6/r  OffSwitchValue=gearoff(10)/3.6/r
  Gear12 : Relay  OnSwitchValue=gearon(11)/3.6/r  OffSwitchValue=gearoff(11)/3.6/r
  Gear13 : Relay  OnSwitchValue=gearon(12)/3.6/r  OffSwitchValue=gearoff(12)/3.6/r
  Gear14 : Relay  OnSwitchValue=gearon(13)/3.6/r  OffSwitchValue=gearoff(13)/3.6/r
  Gear15 : Relay  OnSwitchValue=gearon(14)/3.6/r  OffSwitchValue=gearoff(14)/3.6/r
  Gear16 : Relay  OnSwitchValue=gearon(15)/3.6/r  OffSwitchValue=gearoff(15)/3.6/r
  Gear2 : Relay  OnSwitchValue=gearon(1)/3.6/r  OffSwitchValue=gearoff(1)/3.6/r
  Gear3 : Relay  OnSwitchValue=gearon(2)/3.6/r  OffSwitchValue=gearoff(2)/3.6/r
  Gear4 : Relay  OnSwitchValue=gearon(3)/3.6/r  OffSwitchValue=gearoff(3)/3.6/r
  Gear5 : Relay  OnSwitchValue=gearon(4)/3.6/r  OffSwitchValue=gearoff(4)/3.6/r
  Gear6 : Relay  OnSwitchValue=gearon(5)/3.6/r  OffSwitchValue=gearoff(5)/3.6/r
  Gear7 : Relay  OnSwitchValue=gearon(6)/3.6/r  OffSwitchValue=gearoff(6)/3.6/r
  Gear8 : Relay  OnSwitchValue=gearon(7)/3.6/r  OffSwitchValue=gearoff(7)/3.6/r
  Gear9 : Relay  OnSwitchValue=gearon(8)/3.6/r  OffSwitchValue=gearoff(8)/3.6/r
  Saturation : Saturate  UpperLimit=nog  LowerLimit=0
  Sum : Sum  Inputs=16  SaturateOnIntegerOverflow=on
  Sum1 : Sum  Inputs=2  SaturateOnIntegerOverflow=on
  Gear : Outport
  wires:
  Saturation/1 -> Gear/1
  Gear6/1 -> Sum/6
  Gear7/1 -> Sum/7
  Gear8/1 -> Sum/8
  Gear9/1 -> Sum/9
  Gear10/1 -> Sum/10
  Gear11/1 -> Sum/11
  Gear12/1 -> Sum/12
  Gear13/1 -> Sum/13
  Gear14/1 -> Sum/14
  Gear15/1 -> Sum/15
  Gear16/1 -> Sum/16
  Gear5/1 -> Sum/5
  w_wheel/1 -> Gear16/1, Gear15/1, Gear14/1, Gear13/1, Gear12/1, Gear11/1, Gear10/1, Gear9/1, Gear8/1, Gear7/1, Gear6/1, Gear5/1, Gear1/1, Gear2/1, Gear3/1, Gear4/1
  Gear1/1 -> Sum/1
  Gear2/1 -> Sum/2
  Gear3/1 -> Sum/3
  Gear4/1 -> Sum/4
  Sum/1 -> Sum1/1
  Sum1/1 -> Saturation/1
  Constant/1 -> Sum1/2

== system Chevrolet_PHEVmodel/Automatic Gear Box1/Power flow ==
  w_wheel : Inport
  T_wheel : Inport  Port=2
  gear : Inport  Port=3
  "Engine -> Wheel" : Subsystem
  Saturation : Saturate  UpperLimit=inf  LowerLimit=0
  Switch1 : Switch
  "Wheel -> Engine" : Subsystem
  T_MGB : Outport  InitialOutput=0
  wires:
  w_wheel/1 -> "Wheel -> Engine"/1(w_wheel), "Engine -> Wheel"/1(w_wheel)
  gear/1 -> "Wheel -> Engine"/3(gear), "Engine -> Wheel"/3(gear)
  "Wheel -> Engine"/1(T_MGB-) -> Switch1/3
  Saturation/1 -> "Wheel -> Engine"/2(T_wheel), "Engine -> Wheel"/2(T_wheel), Switch1/2
  "Engine -> Wheel"/1(T_MGB+) -> Switch1/1
  Switch1/1 -> T_MGB/1
  T_wheel/1 -> Saturation/1

== system Chevrolet_PHEVmodel/CE Assignment/Detect fuel cutoff ==
  P_CE_fuel : Inport
  T_CE : Inport  Port=2
  Constant1 : Constant  Value=ENABLE_FUEL_CUTOFF
  Constant3 : Constant  Value=P_CE_cutoff
  Decision : Switch  Threshold=0.5  SaturateOnIntegerOverflow=off  InputSameDT=off
  Detect fuel cutoff : Switch  Threshold=T_CE_cutoff + 0.01
  P_CE : Outport
  wires:
  Constant3/1 -> Detect fuel cutoff/3
  T_CE/1 -> Detect fuel cutoff/2
  P_CE_fuel/1 -> Detect fuel cutoff/1, Decision/3
  Detect fuel cutoff/1 -> Decision/1
  Constant1/1 -> Decision/2
  Decision/1 -> P_CE/1

== system Chevrolet_PHEVmodel/CE Assignment/Detect idle ==
  P_CE_fuel : Inport
  w_CE : Inport  Port=2
  T_CE : Inport  Port=3
  Constant3 : Constant  Value=P_CE_idle
  Idle detection : Fcn  Expr=(u(1) <= w_CE_idle) * (u(2) <= T_CE_idle)
  Mux : Mux  Inputs=2
  Switch2 : Switch  Threshold=0.5
  P_CE : Outport  InitialOutput=0
  wires:
  Mux/1 -> Idle detection/1
  T_CE/1 -> Mux/2
  w_CE/1 -> Mux/1
  Idle detection/1 -> Switch2/2
  P_CE_fuel/1 -> Switch2/3
  Switch2/1 -> P_CE/1
  Constant3/1 -> Switch2/1

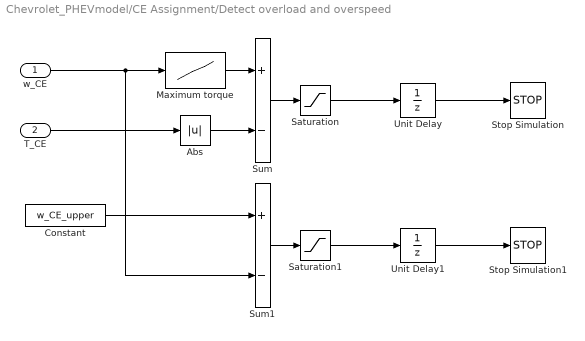
== system Chevrolet_PHEVmodel/CE Assignment/Detect overload and overspeed ==
  w_CE : Inport
  T_CE : Inport  Port=2
  Abs : Abs
  Constant : Constant  Value=w_CE_upper
  Maximum torque : Lookup  InputValues=w_CE_max  Table=T_CE_max
  Saturation : Saturate  UpperLimit=0  LowerLimit=-inf
  Saturation1 : Saturate  UpperLimit=0  LowerLimit=-inf
  Stop Simulation : Stop
  Stop Simulation1 : Stop
  Sum : Sum  Inputs=+-  InputSameDT=on  SaturateOnIntegerOverflow=on  OutDataTypeStr=Inherit: Same as first input
  Sum1 : Sum  Inputs=+-  InputSameDT=on  SaturateOnIntegerOverflow=on  OutDataTypeStr=Inherit: Same as first input
  Unit Delay : UnitDelay  SampleTime=-1  HasFrameUpgradeWarning=on
  Unit Delay1 : UnitDelay  SampleTime=-1  HasFrameUpgradeWarning=on
  wires:
  Sum/1 -> Saturation/1
  w_CE/1 -> Maximum torque/1, Sum1/2
  T_CE/1 -> Abs/1
  Maximum torque/1 -> Sum/1
  Abs/1 -> Sum/2
  Saturation/1 -> Unit Delay/1
  Constant/1 -> Sum1/1
  Sum1/1 -> Saturation1/1
  Saturation1/1 -> Unit Delay1/1
  Unit Delay/1 -> Stop Simulation/1
  Unit Delay1/1 -> Stop Simulation1/1

== system Chevrolet_PHEVmodel/Driving Cycle/Differentiation ==
  V_z : Inport
  Sum1 : Sum  Inputs=+-  InputSameDT=on  SaturateOnIntegerOverflow=on  OutDataTypeStr=Inherit: Same as first input
  Unit Delay1 : UnitDelay  SampleTime=h  HasFrameUpgradeWarning=on
  D_z : Outport  InitialOutput=0
  wires:
  Unit Delay1/1 -> Sum1/2
  V_z/1 -> Sum1/1, Unit Delay1/1
  Sum1/1 -> D_z/1

== system Chevrolet_PHEVmodel/Driving Cycle/Integration ==
  V_z : Inport
  Gain4 : Gain  Gain=0.5*h  SaturateOnIntegerOverflow=on  OutDataTypeStr=Inherit: Same as input  ParamDataTypeStr=Inherit: Same as input
  Plant : UnitDelay  InitialCondition=1  SampleTime=h  HasFrameUpgradeWarning=on
  Sum2 : Sum  InputSameDT=on  SaturateOnIntegerOverflow=on  OutDataTypeStr=Inherit: Same as first input
  Sum4 : Sum  InputSameDT=on  SaturateOnIntegerOverflow=on  OutDataTypeStr=Inherit: Same as first input
  Unit Delay2 : UnitDelay  SampleTime=h  HasFrameUpgradeWarning=on
  x_tot : Outport  InitialOutput=0
  wires:
  Sum2/1 -> Gain4/1
  Unit Delay2/1 -> Sum2/2
  V_z/1 -> Sum2/1, Unit Delay2/1
  Gain4/1 -> Sum4/2
  Sum4/1 -> Plant/1
  Plant/1 -> Sum4/1, x_tot/1

== system Chevrolet_PHEVmodel/EG Assignment/Detect overload and overspeed ==
  w_EG : Inport
  T_EG : Inport  Port=2
  Abs : Abs
  Constant : Constant  Value=w_EG_upper
  Maximum torque : Lookup  InputValues=w_EG_row  Table=T_EG_max
  Saturation : Saturate  UpperLimit=0  LowerLimit=-inf
  Saturation1 : Saturate  UpperLimit=0  LowerLimit=-inf
  Stop Simulation : Stop
  Stop Simulation1 : Stop
  Sum : Sum  Inputs=+-  InputSameDT=on  SaturateOnIntegerOverflow=on  OutDataTypeStr=Inherit: Same as first input
  Sum1 : Sum  Inputs=+-  InputSameDT=on  SaturateOnIntegerOverflow=on  OutDataTypeStr=Inherit: Same as first input
  Unit Delay : UnitDelay  SampleTime=-1  HasFrameUpgradeWarning=on
  Unit Delay1 : UnitDelay  SampleTime=-1  HasFrameUpgradeWarning=on
  wires:
  Saturation1/1 -> Unit Delay1/1
  Sum1/1 -> Saturation1/1
  Constant/1 -> Sum1/1
  Saturation/1 -> Unit Delay/1
  Abs/1 -> Sum/2
  Maximum torque/1 -> Sum/1
  T_EG/1 -> Abs/1
  w_EG/1 -> Sum1/2, Maximum torque/1
  Sum/1 -> Saturation/1
  Unit Delay/1 -> Stop Simulation/1
  Unit Delay1/1 -> Stop Simulation1/1

== system Chevrolet_PHEVmodel/EM Assignment/Detect overload and overspeed ==
  w_EM : Inport
  T_EM : Inport  Port=2
  Abs : Abs
  Constant : Constant  Value=w_EM_upper
  Maximum torque : Lookup  InputValues=w_EM_row  Table=T_EM_max
  Saturation : Saturate  UpperLimit=0  LowerLimit=-inf
  Saturation1 : Saturate  UpperLimit=0  LowerLimit=-inf
  Stop Simulation : Stop
  Stop Simulation1 : Stop
  Sum : Sum  Inputs=+-  InputSameDT=on  SaturateOnIntegerOverflow=on  OutDataTypeStr=Inherit: Same as first input
  Sum1 : Sum  Inputs=+-  InputSameDT=on  SaturateOnIntegerOverflow=on  OutDataTypeStr=Inherit: Same as first input
  Unit Delay : UnitDelay  SampleTime=-1  HasFrameUpgradeWarning=on
  Unit Delay1 : UnitDelay  SampleTime=-1  HasFrameUpgradeWarning=on
  wires:
  Sum/1 -> Saturation/1
  w_EM/1 -> Maximum torque/1, Sum1/2
  T_EM/1 -> Abs/1
  Maximum torque/1 -> Sum/1
  Abs/1 -> Sum/2
  Saturation/1 -> Unit Delay/1
  Constant/1 -> Sum1/1
  Sum1/1 -> Saturation1/1
  Saturation1/1 -> Unit Delay1/1
  Unit Delay/1 -> Stop Simulation/1
  Unit Delay1/1 -> Stop Simulation1/1

== system Chevrolet_PHEVmodel/PHEV Battery/Cell electrical model ==
  I_cell [A] : Inport
  Rt_initSOC [-] : Inport  Port=2
  Add3 : Sum
  DOD->SOC : Fcn  Expr=1-u(1)
  Open-circuit voltage : Lookup  InputValues=[-0.08,-0.03,0,0.005,0.025,0.05,0.085,0.155,0.25,0.3,0.34,0.365,0.395,0.41,0.5,0.52,0.62,0.7,0.73,0.76,0.8,0.82,0.83,0.85,0.89,0.9,0.91,0.92,0.935,0.95,0.965,0.98,0.99,0.995,1,1.011,1.015]  Table=[4.32,4.22,4.15,4.12,4.115,4.1,4.07,4.03,3.96,3.92,3.915,3.8937,3.8622,3.8537,3.7828,3.7672,3.7022,3.6562,3.6398,3.6098,3.4,3.3,3.2,3.18,3.17,3.15,3.1,3.1,3,2.95,2.8437,2.8437,2.8437,2.8437,2.8437,2.5,2]  LookUpMeth=Interpolation-Use End Values  SaturateOnIntegerOverflow=off
  Product1 : Product  Inputs=**  RndMeth=Zero
  Product2 : Product  Inputs=**  RndMeth=Zero
  Resistance : Lookup  InputValues=[0,0.16666666666666666,0.3333333333333333,0.5,0.6666666666666666,0.8333333333333334,1]  Table=0.5*[0.024012,0.0100,0.0075,0.00375,0.0022500000000000003,0.0015,0.0011250000000000001]  SaturateOnIntegerOverflow=off
  State of charge calculation : Subsystem
  Stop Function : Subsystem
  Rt_SOC [-] : Outport
  U_cell [V] : Outport  Port=2
  Pw_CellLoss : Outport  Port=3
  wires:
  State of charge calculation/1(Rt_SOC [-]) -> Rt_SOC [-]/1
  State of charge calculation/2(Rt_DOD [-]) -> DOD->SOC/1, Open-circuit voltage/1
  Open-circuit voltage/1 -> Add3/1
  Add3/1 -> Stop Function/3(U_Cell), U_cell [V]/1
  Rt_initSOC [-]/1 -> State of charge calculation/2(Rt_initSOC [-])
  Product2/1 -> Product1/1, Add3/2  "U_DropCell"
  I_cell [A]/1 -> Stop Function/1(I_cell [A]), Product2/2, Product1/2, State of charge calculation/1(I_cell [A])
  Resistance/1 -> Product2/1
  DOD->SOC/1 -> Stop Function/2(Rt_SOC), Resistance/1
  Product1/1 -> Pw_CellLoss/1  "Pw_LossCell"

== system Chevrolet_PHEVmodel/Tank/Integration ==
  P_fuel : Inport
  Constant : Constant  Value=1/H_u
  Fuel consumption : UnitDelay  SampleTime=h  HasFrameUpgradeWarning=on
  Gain3 : Gain  Gain=.5*h  SaturateOnIntegerOverflow=on  OutDataTypeStr=Inherit: Same as input  ParamDataTypeStr=Inherit: Same as input
  Product2 : Product  InputSameDT=on  RndMeth=Zero  SaturateOnIntegerOverflow=on  OutDataTypeStr=Inherit: Same as first input
  Sum1 : Sum  InputSameDT=on  SaturateOnIntegerOverflow=on  OutDataTypeStr=Inherit: Same as first input
  Sum4 : Sum  InputSameDT=on  SaturateOnIntegerOverflow=on  OutDataTypeStr=Inherit: Same as first input
  To Workspace1 : ToWorkspace  VariableName=m_dot_fuel  SampleTime=-1
  To Workspace2 : ToWorkspace  VariableName=m_fuel  SampleTime=-1
  Unit Delay3 : UnitDelay  SampleTime=h  HasFrameUpgradeWarning=on
  m_fuel : Outport  InitialOutput=0
  wires:
  Product2/1 -> To Workspace1/1, Sum4/2
  Sum4/1 -> Fuel consumption/1
  Fuel consumption/1 -> To Workspace2/1, Sum4/1, m_fuel/1
  Sum1/1 -> Gain3/1
  Unit Delay3/1 -> Sum1/2
  P_fuel/1 -> Unit Delay3/1, Sum1/1
  Gain3/1 -> Product2/2
  Constant/1 -> Product2/1

== system Chevrolet_PHEVmodel/Vehicle/Acceleration Force ==
  a_veh : Inport
  Inertia : Fcn  Expr=m_f*u/h
  F_Net : Outport  InitialOutput=0
  wires:
  a_veh/1 -> Inertia/1
  Inertia/1 -> F_Net/1

== system Chevrolet_PHEVmodel/Vehicle/Aerodynamic resistance ==
  v : Inport
  Aerodynamic resistance : Fcn  Expr=0.5*rho*cw*A_f*u^2
  F_aero : Outport  InitialOutput=0
  wires:
  Aerodynamic resistance/1 -> F_aero/1
  v/1 -> Aerodynamic resistance/1

== system Chevrolet_PHEVmodel/Vehicle/Average speed ==
  v : Inport
  Gain5 : Gain  Gain=0.5  SaturateOnIntegerOverflow=on  OutDataTypeStr=Inherit: Same as input  ParamDataTypeStr=Inherit: Same as input
  Sum2 : Sum  InputSameDT=on  SaturateOnIntegerOverflow=on  OutDataTypeStr=Inherit: Same as first input
  Unit Delay : UnitDelay  SampleTime=-1  HasFrameUpgradeWarning=on
  v_a : Outport  InitialOutput=0
  wires:
  Unit Delay/1 -> Sum2/2
  Sum2/1 -> Gain5/1
  Gain5/1 -> v_a/1
  v/1 -> Sum2/1, Unit Delay/1

== system Chevrolet_PHEVmodel/Vehicle/Rolling resistance ==
  v : Inport
  alfa : Inport  Port=2
  Inertia : Fcn  Expr=m_f*g*mu*cos(u)
  Switch : Switch  Criteria=u2 > Threshold  Threshold=eps  SaturateOnIntegerOverflow=off  InputSameDT=off
  standstill : Constant  Value=0
  F_roll : Outport
  wires:
  Inertia/1 -> Switch/1
  standstill/1 -> Switch/3
  v/1 -> Switch/2
  Switch/1 -> F_roll/1
  alfa/1 -> Inertia/1

== system Chevrolet_PHEVmodel/Vehicle/gradient force ==
  alfa : Inport
  grade : Fcn  Expr=m_f*g*sin(u)
  F_grade : Outport  InitialOutput=0
  wires:
  grade/1 -> F_grade/1
  alfa/1 -> grade/1

== system Chevrolet_PHEVmodel/Automatic Gear Box/Power flow/Engine -> Wheel ==
  w_wheel : Inport
  T_wheel : Inport  Port=2
  gear : Inport  Port=3
  Constant1 : Constant  Value=P_GT0
  Constant2 : Constant  Value=inf
  Gain : Gain  Gain=e_GT  SaturateOnIntegerOverflow=on  OutDataTypeStr=Inherit: Same as input  ParamDataTypeStr=Inherit: Same as input
  Product2 : Product  Inputs=*/  InputSameDT=on  RndMeth=Zero  SaturateOnIntegerOverflow=on  OutDataTypeStr=Inherit: Same as first input
  Product3 : Product  Inputs=/*  InputSameDT=on  RndMeth=Zero  SaturateOnIntegerOverflow=on  OutDataTypeStr=Inherit: Same as first input
  Sum : Sum  InputSameDT=on  SaturateOnIntegerOverflow=on  OutDataTypeStr=Inherit: Same as first input
  Switch1 : Switch  Threshold=w_wheel_min
  T_MGB+ : Outport  InitialOutput=0
  wires:
  T_wheel/1 -> Sum/2
  Product3/1 -> Sum/1
  Gain/1 -> Product2/2
  Product2/1 -> T_MGB+/1
  Sum/1 -> Product2/1
  w_wheel/1 -> Switch1/2, Switch1/1
  Constant2/1 -> Switch1/3
  Switch1/1 -> Product3/1
  Constant1/1 -> Product3/2
  gear/1 -> Gain/1

== system Chevrolet_PHEVmodel/Automatic Gear Box/Power flow/Wheel -> Engine ==
  w_wheel : Inport
  T_wheel : Inport  Port=2
  gear : Inport  Port=3
  Constant1 : Constant  Value=P_GT0
  Constant2 : Constant  Value=inf
  Gain1 : Gain  Gain=e_GT  SaturateOnIntegerOverflow=on  OutDataTypeStr=Inherit: Same as input  ParamDataTypeStr=Inherit: Same as input
  Gain2 : Gain  Gain=1/e_GT  SaturateOnIntegerOverflow=on  OutDataTypeStr=Inherit: Same as input  ParamDataTypeStr=Inherit: Same as input
  Product2 : Product  Inputs=*/  InputSameDT=on  RndMeth=Zero  SaturateOnIntegerOverflow=on  OutDataTypeStr=Inherit: Same as first input
  Product3 : Product  Inputs=/*  InputSameDT=on  RndMeth=Zero  SaturateOnIntegerOverflow=on  OutDataTypeStr=Inherit: Same as first input
  Sum : Sum  InputSameDT=on  SaturateOnIntegerOverflow=on  OutDataTypeStr=Inherit: Same as first input
  Switch1 : Switch  Threshold=w_wheel_min
  T_MGB- : Outport  InitialOutput=0
  wires:
  w_wheel/1 -> Switch1/1, Switch1/2
  gear/1 -> Gain2/1
  Constant2/1 -> Switch1/3
  Switch1/1 -> Gain1/1
  Constant1/1 -> Product3/2
  T_wheel/1 -> Sum/1
  Gain2/1 -> Product2/2
  Product2/1 -> T_MGB-/1
  Product3/1 -> Sum/2
  Sum/1 -> Product2/1
  Gain1/1 -> Product3/1

== system Chevrolet_PHEVmodel/Automatic Gear Box1/Power flow/Engine -> Wheel ==
  w_wheel : Inport
  T_wheel : Inport  Port=2
  gear : Inport  Port=3
  Constant1 : Constant  Value=P_GT0
  Constant2 : Constant  Value=inf
  Gain : Gain  Gain=e_GT  SaturateOnIntegerOverflow=on  OutDataTypeStr=Inherit: Same as input  ParamDataTypeStr=Inherit: Same as input
  Product2 : Product  Inputs=*/  InputSameDT=on  RndMeth=Zero  SaturateOnIntegerOverflow=on  OutDataTypeStr=Inherit: Same as first input
  Product3 : Product  Inputs=/*  InputSameDT=on  RndMeth=Zero  SaturateOnIntegerOverflow=on  OutDataTypeStr=Inherit: Same as first input
  Sum : Sum  InputSameDT=on  SaturateOnIntegerOverflow=on  OutDataTypeStr=Inherit: Same as first input
  Switch1 : Switch  Threshold=w_wheel_min
  T_MGB+ : Outport  InitialOutput=0
  wires:
  T_wheel/1 -> Sum/2
  Product3/1 -> Sum/1
  Gain/1 -> Product2/2
  Product2/1 -> T_MGB+/1
  Sum/1 -> Product2/1
  w_wheel/1 -> Switch1/2, Switch1/1
  Constant2/1 -> Switch1/3
  Switch1/1 -> Product3/1
  Constant1/1 -> Product3/2
  gear/1 -> Gain/1
